simulink model "multichanel_framebased"  (R2024a)
settings: Solver=FixedStepDiscrete  StartTime=0.0  StopTime=inf  RelTol=1e-3
libraries: dspsrcs4 x2, dspsnks4 x1, dspvision x1
settings Model: Creator=Admin  LastModifiedBy=Admin

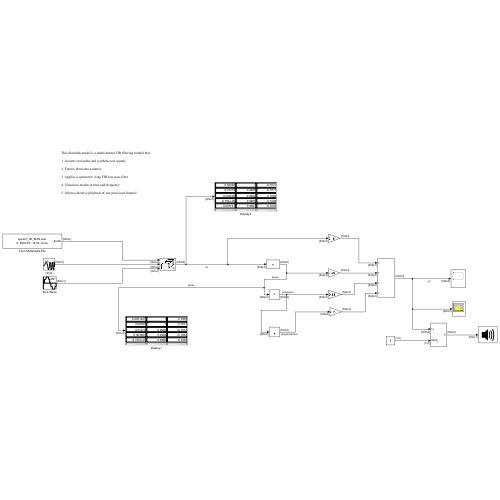
[thumbnail: Simulink's stored preview of the top-level diagram]
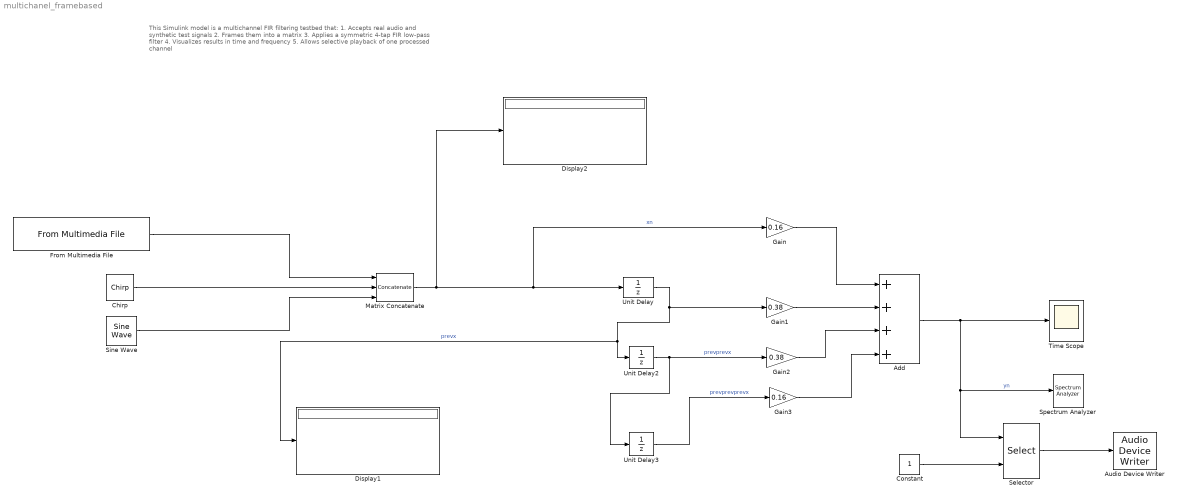
== system multichanel_framebased ==
  note: This Simulink model is a multichannel FIR filtering testbed that:
      |
      | 1. Accepts real audio and synthetic test signals
      |
      | 2. Frames them into a matrix
      |
      | 3. Applies a symmetric 4-tap FIR low-pass filter
      |
      | 4. Visualizes results in time and frequency
      |
      | 5. Allows selective playback of one processed channel
  Add : Sum  Inputs=++++
  Audio Device Writer : dspsnks4/Audio Device Writer  Driver=DirectSound  Device=Default  InheritSampleRate=on  SampleRate=44100  BitDepth=16-bit integer  BufferSize=4096  NumBuffers=10  DefaultOutputChannelMapping=on  OutputChannelMapping=1:2  OutputNumUnderrunSamples=off  DriverIdx=1  DeviceWarnFlag=''
  Chirp : dspsrcs4/Chirp  sweep=Linear  mode=Bidirectional  f0=0  f1=25  t1=1  Tsweep=1  phase=pi/2  Ts=1/8000  spf=500  datatype=double  OutputFrames=off
  Constant : Constant  VectorParams1D=off
  Display1 : Display
  Display2 : Display
  From Multimedia File : dspvision/From Multimedia File  inputFilename=C:\Program Files\MATLAB\R2024a\toolbox\dsp\dsp\samples\speech_dft_8kHz.wav  readRange=[1 Inf]  loop=on  numPlays=inf  outputStreams=Audio only  videoDataType=single  audioDataType=double  inheritSampleTime=on  userDefinedSampleTime=1/30  noAudioOutput=off  isIntensityVideo=off  fourcc=RGB  colorVideoFormat=One multidimensional signal  outputEOF=off  dataOrg=Column-major  audioFrameSize=500  computeAudioFrameSize=off  outSamplingMode=Sample based
      settings: LibrarySourceBlock=dspsrcs4/From Multimedia File
  Gain : Gain  Gain=0.16
  Gain1 : Gain  Gain=0.38
  Gain2 : Gain  Gain=0.38
  Gain3 : Gain  Gain=0.16
  Matrix Concatenate : Concatenate  NumInputs=3  Mode=Multidimensional array  ConcatenateDimension=2
  Selector : Selector  NumberOfDimensions=2  InputPortWidth=3  IndexOptions=Select all,Index vector (port)  Indices=[1 3],1  OutputSizes=1,1
  Sine Wave : dspsrcs4/Sine Wave  Amplitude=1  Frequency=1  Phase=0  SampleMode=Discrete  OutComplex=Real  CompMethod=Trigonometric fcn  TableSize=Speed  SampleTime=1/8000  SamplesPerFrame=500  ResetState=Restart at time zero  OutputFrames=off  dataType=double  wordLen=16  udDataType=sfix(16)  fracBitsMode=Best precision  numFracBits=15  OutDataTypeStr=double  LastOutDataTypeStr=double
  Spectrum Analyzer : SpectrumAnalyzer  WindowPosition=[1.000000,141.000000,650.000000,403.000000,]  ScopeFrameLocation=window  Span=8000  StartFrequency=-4000  StopFrequency=4000  YLimits=[-190.6432099,51.80879399]
  Time Scope : Scope
  Unit Delay : UnitDelay  InputProcessing=Columns as channels (frame based)  SampleTime=-1  HasFrameUpgradeWarning=on
  Unit Delay2 : UnitDelay  InputProcessing=Columns as channels (frame based)  SampleTime=-1  HasFrameUpgradeWarning=on
  Unit Delay3 : UnitDelay  InputProcessing=Columns as channels (frame based)  SampleTime=-1  HasFrameUpgradeWarning=on
  wires:
  From Multimedia File/1 -> Matrix Concatenate/1
  Chirp/1 -> Matrix Concatenate/2
  Sine Wave/1 -> Matrix Concatenate/3
  Matrix Concatenate/1 -> Display2/1, Gain/1, Unit Delay/1  "xn"
  Unit Delay/1 -> Unit Delay2/1, Display1/1, Gain1/1  "prevx"
  Unit Delay3/1 -> Gain3/1  "prevprevprevx"
  Unit Delay2/1 -> Gain2/1, Unit Delay3/1  "prevprevx"
  Gain/1 -> Add/1
  Gain1/1 -> Add/2
  Gain2/1 -> Add/3
  Gain3/1 -> Add/4
  Add/1 -> Spectrum Analyzer/1, Selector/1, Time Scope/1  "yn"
  Selector/1 -> Audio Device Writer/1
  Constant/1 -> Selector/2
